simulink model "chap11_2sim"  (Simulink 5.0)
settings: Solver=ode45  StartTime=0.0  StopTime=1  FixedStep=0.001  RelTol=1e-8  AbsTol=1e-8
PreLoadFcn:
  | i=k;
values from neighbouring files (symbols this model uses):
  k = k'    [chap11_1main.m]    (also in chap11_2main.m)
libraries: simulink x1
settings Model: LastModifiedBy=Administrator  MaxDataPoints=10000  RTWOptions="-aEnforceIntegerDowncast=1 -aExtMode=0 -aExtModeTesting=0 -aFoldNonRolledExpr=1 -aForceParamTrailComments=0 -aGenerateComments=1 -aGenerateReport=0 -aIgnoreCustomStorageClasses=1 -aIncDataTypeInIds=0 -aIncHierarchyInIds=0 -aInlineInvariantSignals=0 -aInlinedPrmAccess=\"Literals\" -aLocalBlockOutputs=1 -aLogVarNameModifier=\"rt_\" -aMaxRTWIdLen=31 -aPrefixModelToSubsysFcnNames=1 -aRTWVerbose=1 -aRollThreshold=5 -aShowEliminatedStatements=0"

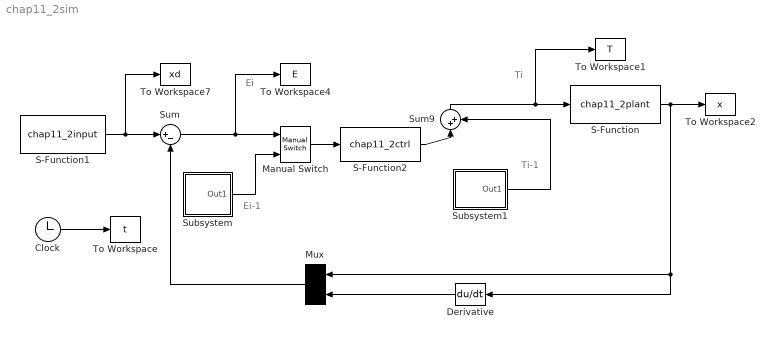
== system chap11_2sim ==
  note: Ti
  note: Ti-1
  note: Ei
  note: Ei-1
  Clock : Clock
      settings: Decimation=10
  Derivative : Derivative  Orientation=left
  Manual Switch : simulink/Signal Routing/Manual Switch  sw=1  action=0
  Mux : Mux  Orientation=left  Inputs=2
  S-Function : S-Function  FunctionName=chap11_2plant
  S-Function1 : S-Function  FunctionName=chap11_2input
  S-Function2 : S-Function  FunctionName=chap11_2ctrl
  Subsystem : Subsystem
  Subsystem1 : Subsystem
  Sum : Sum  Inputs=|+-  SaturateOnIntegerOverflow=on
  Sum9 : Sum  Orientation=up  Inputs=|++  SaturateOnIntegerOverflow=on
  To Workspace : ToWorkspace  VariableName=t  SampleTime=-1  SaveFormat=Array
  To Workspace1 : ToWorkspace  VariableName=T  SampleTime=-1  SaveFormat=Array
  To Workspace2 : ToWorkspace  VariableName=x  SampleTime=-1  SaveFormat=Array
  To Workspace4 : ToWorkspace  VariableName=E  SampleTime=-1  SaveFormat=Array
  To Workspace7 : ToWorkspace  VariableName=xd  SampleTime=-1  SaveFormat=Array
  wires:
  S-Function/1 -> To Workspace2/1, Derivative/1, Mux/1
  Clock/1 -> To Workspace/1
  S-Function1/1 -> To Workspace7/1, Sum/1
  S-Function2/1 -> Sum9/1
  Sum9/1 -> S-Function/1, To Workspace1/1
  Subsystem1/1(Out1) -> Sum9/2
  Sum/1 -> To Workspace4/1, Manual Switch/1
  Derivative/1 -> Mux/2
  Mux/1 -> Sum/2
  Manual Switch/1 -> S-Function2/1
  Subsystem/1(Out1) -> Manual Switch/2

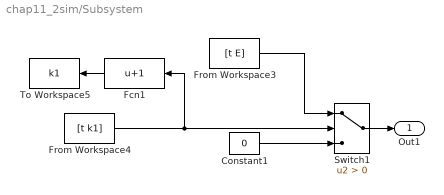
== system chap11_2sim/Subsystem ==
  Constant1 : Constant  Value=0
  Fcn1 : Fcn  Orientation=left  Expr=u+1
  From Workspace3 : FromWorkspace  VariableName=[t E]  SampleTime=0
  From Workspace4 : FromWorkspace  VariableName=[t k1]  SampleTime=0
  Switch1 : Switch  Criteria=u2 > Threshold  SaturateOnIntegerOverflow=on
  To Workspace5 : ToWorkspace  VariableName=k1  SampleTime=-1  SaveFormat=Array
  Out1 : Outport
  wires:
  Constant1/1 -> Switch1/3
  From Workspace3/1 -> Switch1/1
  From Workspace4/1 -> Fcn1/1, Switch1/2
  Fcn1/1 -> To Workspace5/1
  Switch1/1 -> Out1/1

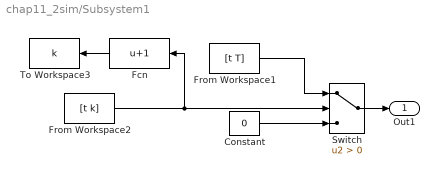
== system chap11_2sim/Subsystem1 ==
  Constant : Constant  Value=0
  Fcn : Fcn  Orientation=left  Expr=u+1
  From Workspace1 : FromWorkspace  VariableName=[t T]  SampleTime=0
  From Workspace2 : FromWorkspace  VariableName=[t k]  SampleTime=0
  Switch : Switch  Criteria=u2 > Threshold  SaturateOnIntegerOverflow=on
  To Workspace3 : ToWorkspace  VariableName=k  SampleTime=-1  SaveFormat=Array
  Out1 : Outport
  wires:
  Constant/1 -> Switch/3
  From Workspace1/1 -> Switch/1
  From Workspace2/1 -> Fcn/1, Switch/2
  Fcn/1 -> To Workspace3/1
  Switch/1 -> Out1/1
